simulink subsystem "LiftPlusCruise"  (R2022b)
settings: Solver=VariableStepAuto  StartTime=0.0  StopTime=10.0  RelTol=1e-3
settings Model: Creator=tbritton  LastModifiedBy=macheson
settings SolverCC: AlgebraicLoopSolver=TrustRegion
settings DebuggingCC: UnconnectedInputMsg=warning  UnconnectedOutputMsg=warning  UnconnectedLineMsg=warning  SFMachineParentedDataDiag=warning
settings ModelReferenceCC: EnableRefExpFcnMdlSchedulingChecks=on
settings RTWCC: DLArmComputeVersion=19.05

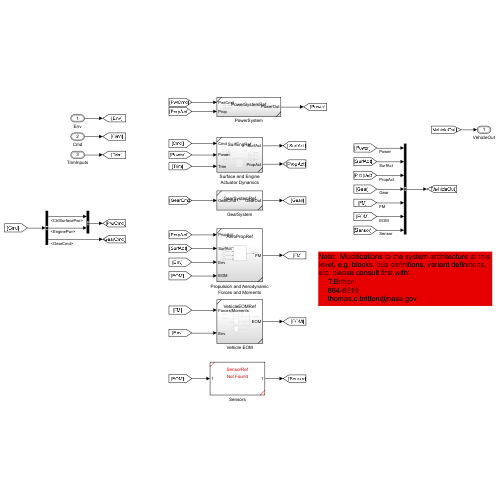
[thumbnail: Simulink's stored preview of the top-level diagram]
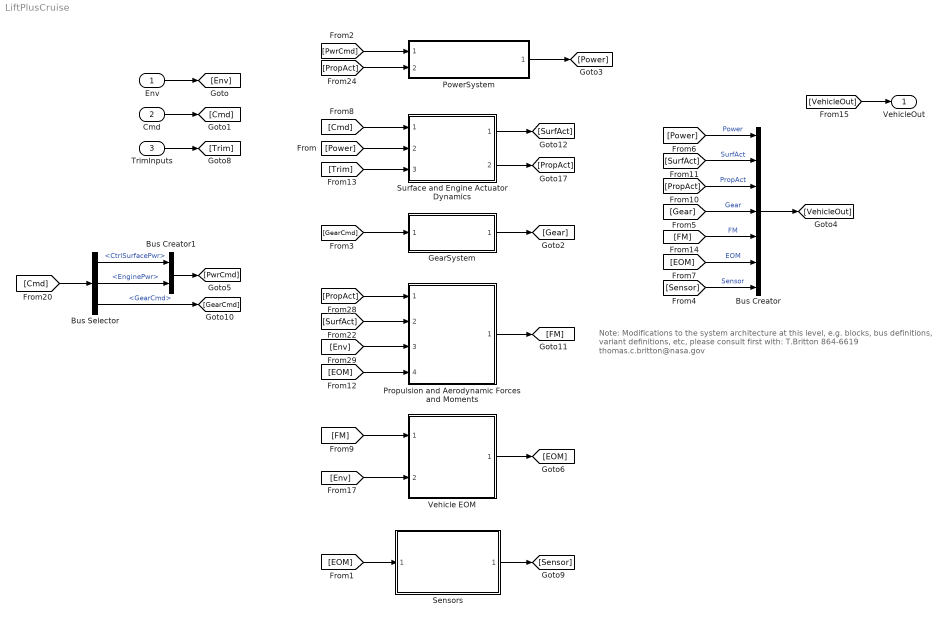
== system LiftPlusCruise ==
  note: Note: Modifications to the system architecture at this level, e.g. blocks, bus definitions, variant definitions, etc, please consult first with:
      | T.Britton
      | 864-6619
      | thomas.c.britton@nasa.gov
  Env : Inport  OutDataTypeStr=Bus: EnvironmentBus
  Cmd : Inport  Port=2  OutDataTypeStr=Bus: BUS_CMD
  TrimInputs : Inport  Port=3  OutDataTypeStr=Bus: BUS_TRIM_INPUT
  Bus Creator : BusCreator  Inputs=7  OutDataTypeStr=Bus: BUS_VEHICLE_OUT
  Bus Creator1 : BusCreator  Inputs=2  OutDataTypeStr=Bus: BUS_POWER_SYSTEM_IN
  Bus Selector : BusSelector  OutputSignals=CtrlSurfacePwr,EnginePwr,GearCmd
  GearSystem : Subsystem  ReferencedSubsystem=GearSystemRef
  PowerSystem : Subsystem  ReferencedSubsystem=PowerSystemRef
  Propulsion and Aerodynamic Forces and Moments : Subsystem  ReferencedSubsystem=AeroPropRef
  Sensors : Subsystem  ReferencedSubsystem=SensorRef
  Surface and Engine Actuator Dynamics : Subsystem  ReferencedSubsystem=SurfEngRef
  Vehicle EOM : Subsystem  ReferencedSubsystem=VehicleEOMRef
  "VehicleOut " : Outport  OutDataTypeStr=Bus: BUS_VEHICLE_OUT  VectorParamsAs1DForOutWhenUnconnected=off
  wires:
  [VehicleOut] -> "VehicleOut "/1
  Bus Creator/1 -> [VehicleOut]
  [Sensor] -> Bus Creator/7  "Sensor"
  [EOM] -> Bus Creator/6  "EOM"
  [FM] -> Bus Creator/5  "FM"
  [PropAct] -> Bus Creator/3  "PropAct"
  [Gear] -> Bus Creator/4  "Gear"
  [SurfAct] -> Bus Creator/2  "SurfAct"
  [Power] -> Bus Creator/1  "Power"
  Surface and Engine Actuator Dynamics/2 -> [PropAct]
  Surface and Engine Actuator Dynamics/1 -> [SurfAct]
  [Trim] -> Surface and Engine Actuator Dynamics/3
  [Power] -> Surface and Engine Actuator Dynamics/2
  [Cmd] -> Surface and Engine Actuator Dynamics/1
  [Env] -> Vehicle EOM/2
  Vehicle EOM/1 -> [EOM]
  [FM] -> Vehicle EOM/1
  TrimInputs/1 -> [Trim]
  Bus Creator1/1 -> [PwrCmd]
  Bus Selector/2 -> Bus Creator1/2  "<EnginePwr>"
  [Cmd] -> Bus Selector/1
  [GearCmd] -> GearSystem/1
  Env/1 -> [Env]
  Cmd/1 -> [Cmd]
  GearSystem/1 -> [Gear]
  PowerSystem/1 -> [Power]
  [PwrCmd] -> PowerSystem/1
  Bus Selector/3 -> [GearCmd]  "<GearCmd>"
  Bus Selector/1 -> Bus Creator1/1  "<CtrlSurfacePwr>"
  [PropAct] -> PowerSystem/2
  [PropAct] -> Propulsion and Aerodynamic Forces and Moments/1
  [SurfAct] -> Propulsion and Aerodynamic Forces and Moments/2
  [Env] -> Propulsion and Aerodynamic Forces and Moments/3
  [EOM] -> Propulsion and Aerodynamic Forces and Moments/4
  Propulsion and Aerodynamic Forces and Moments/1 -> [FM]
  [EOM] -> Sensors/1
  Sensors/1 -> [Sensor]
